simulink model "malt_pos_hold"  (R2023a)
settings: Solver=FixedStepAuto  StartTime=0.0  StopTime=50  FixedStep=framePeriod_s  RelTol=1e-3
undefined symbols (not defined in the file or in its folder): Aircraft, DiscIntNeverNeededParam, framePeriod_s, frameRate_hz
libraries: simulink x33, slpidlib x12
(part 2 of 3)

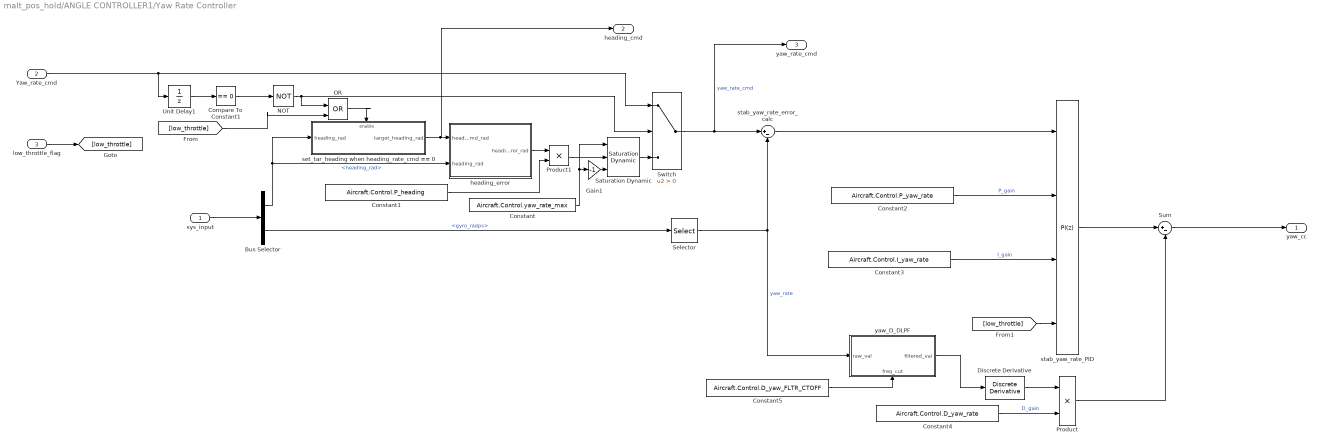
== system malt_pos_hold/ANGLE CONTROLLER1/Yaw Rate Controller ==
  sys_input : Inport
  Yaw_rate_cmd : Inport  Port=2
  low_throttle_flag : Inport  Port=3
  Bus Selector : BusSelector  OutputSignals=StateEstData.bfs_ins.heading_rad,StateEstData.bfs_ins.gyro_radps
  Compare To Constant1 : simulink/Logic and Bit Operations/Compare To Constant  relop===  const=0  OutDataTypeStr=boolean
  Constant : Constant  Value=Aircraft.Control.yaw_rate_max
  Constant1 : Constant  Value=Aircraft.Control.P_heading  OutDataTypeStr=single
  Constant2 : Constant  Value=Aircraft.Control.P_yaw_rate  OutDataTypeStr=single
  Constant3 : Constant  Value=Aircraft.Control.I_yaw_rate  OutDataTypeStr=single
  Constant4 : Constant  Value=Aircraft.Control.D_yaw_rate  OutDataTypeStr=single
  Constant5 : Constant  Value=Aircraft.Control.D_yaw_FLTR_CTOFF  OutDataTypeStr=single
  Discrete Derivative : simulink/Quick Insert/Discrete/Discrete Derivative  gainval=1.0  ICPrevScaledInput=0.0  OutMin=[]  OutMax=[]  OutDataType=fixdt(1, 16)  OutScaling=2^-10  DoSatur=off
  Gain1 : Gain  Gain=-1
  NOT : Logic  Operator=NOT  IconShape=distinctive  AllPortsSameDT=off  OutDataTypeStr=boolean
  OR : Logic  Operator=OR  IconShape=distinctive  AllPortsSameDT=off  OutDataTypeStr=boolean
  Product : Product
  Product1 : Product
  Saturation Dynamic : simulink/Discontinuities/Saturation Dynamic  OutMin=[]  OutMax=[]  OutDataTypeStr=Inherit: Same as second input  OutDataType=fixdt(1, 16)  OutScaling=2^-10  DoSatur=off
  Selector : Selector  InputPortWidth=3  IndexOptions=Index vector (dialog)  Indices=3  OutputSizes=1
  Sum : Sum  Inputs=|+-
  Switch : Switch  Criteria=u2 > Threshold  SaturateOnIntegerOverflow=off  InputSameDT=off
  Unit Delay1 : UnitDelay  InitialCondition=0.5  SampleTime=-1  HasFrameUpgradeWarning=on
  heading_error : Subsystem
  set_tar_heading when heading_rate_cmd == 0 : Subsystem  TreatAsAtomicUnit=on
  stab_yaw_rate_PID : slpidlib/PID Controller  Controller=PI  Form=Parallel  TimeDomain=Discrete-time  UseExternalTs=off  SampleTime=framePeriod_s  IntegratorMethod=Forward Euler  FilterMethod=Forward Euler  ControllerParametersSource=external  P=1.85  I=0.01  UseKiTs=off  D=0  N=100  UseFilter=off  TunerSelectOption=Transfer Function Based (PID Tuner App)  InitialConditionSource=internal  InitialConditionForIntegrator=0  InitialConditionForFilter=0  DifferentiatorICPrevScaledInput=0  ExternalReset=either  TrackingMode=off  Kt=1  LimitOutput=on  SatLimitsSource=internal  UpperSaturationLimit=1  LowerSaturationLimit=-1  LinearizeAsGain=off  AntiWindupMode=clamping  Kb=1  LimitIntegrator=off  UpperIntegratorSaturationLimit=inf  LowerIntegratorSaturationLimit=-inf  POutMin=[]  POutMax=[]  IOutMin=[]  IOutMax=[]  DOutMin=[]  DOutMax=[]  NOutMin=[]  NOutMax=[]  SumOutMin=[]  SumOutMax=[]  SaturationOutMin=[]  SaturationOutMax=[]  PParamMin=[]  PParamMax=[]  IParamMin=[]  IParamMax=[]  DParamMin=[]  DParamMax=[]  NParamMin=[]  NParamMax=[]  KbParamMin=[]  KbParamMax=[]  KtParamMin=[]  KtParamMax=[]  KbOutMin=[]  KbOutMax=[]  KtOutMin=[]  KtOutMax=[]  IntegratorOutMin=[]  IntegratorOutMax=[]  FilterOutMin=[]  FilterOutMax=[]  SumI1OutMin=[]  SumI1OutMax=[]  SumI2OutMin=[]  SumI2OutMax=[]  SumI3OutMin=[]  SumI3OutMax=[]  SumI4OutMin=[]  SumI4OutMax=[]  SumDOutMin=[]  SumDOutMax=[]  DifferentiatorOutMin=[]  DifferentiatorOutMax=[]  FilterDiffOutCoefMin=[]  FilterDiffOutCoefMax=[]  ReciprocalOutMin=[]  ReciprocalOutMax=[]  SumDenOutMin=[]  SumDenOutMax=[]  SumNumOutMin=[]  SumNumOutMax=[]  DivideOutMin=[]  DivideOutMax=[]  UdiffTsProdOutMin=[]  UdiffTsProdOutMax=[]  NTsProdOutMin=[]  NTsProdOutMax=[]  UintegralTsProdOutMin=[]  UintegralTsProdOutMax=[]  UngainTsProdOutMin=[]  UngainTsProdOutMax=[]  ClampingZeroOutDataTypeStr=Inherit: Inherit via back propagation  ClampingZeroOutMin=[]  ClampingZeroOutMax=[]  FilterDenConstantOutDataTypeStr=Inherit: Inherit via back propagation  FilterDenConstantOutMin=[]  FilterDenConstantOutMax=[]  PCopyOutDataTypeStr=Inherit: Inherit via back propagation  PCopyOutMin=[]  PCopyOutMax=[]  NCopyOutDataTypeStr=Inherit: Inherit via back propagation  NCopyOutMin=[]  NCopyOutMax=[]  IntegratorContinuousStateAttributes=''  IntegratorStateMustResolveToSignalObject=off  IntegratorRTWStateStorageClass=Auto  FilterContinuousStateAttributes=''  FilterStateMustResolveToSignalObject=off  FilterRTWStateStorageClass=Auto  ParallelPVariant=ExternalParameters  IdealPVariant=Disabled  IVariant=ExternalParameters  DVariant=Disabled  IntegratorVariant=Discrete  SatVariant=Enabled  AWVariant=DiscClampingParallel  PCopyVariant=Disabled  TRVariant=Disabled  FdbkBlocksVariant=Forward  IdealPFdbkVariant=Disabled  SatFdbkVariant=Disabled  DerivativeFilterVariant=Disabled  NVariant=Disabled  NCopyVariant=Disabled_SignalSpec  FilterICVariant=Disabled  IntegratorICVariant=InternalICs  ExternalResetVariant=ExternalReset  TRSumVariant=Passthrough  SumFdbkVariant=Disabled  SumVariant=Sum_PI  TsampFilterVariant=InternalTs  TsampNgainVariant=Passthrough  TsampIntegralVariant=Disabled_SignalSpec  ExternalSaturationOutDataTypeStr=Inherit: Same as second input
  stab_yaw_rate_error_calc : Sum  Inputs=|+-
  yaw_D_DLPF : Subsystem
      settings: PortSchema="{\"entries\":[{\"content\":{\"sides\":[{\"content\":{\"connectorIds\":[\"In1\"]},\"type\":\"ConnectorPlacement.EquallySpacedRectSide\",\"uuid\":\"20236834-aeb3-4c5b-bb2e-f84447e752b5\"},{\"content\":{\"connectorIds\":[\"Out1\"],\"side\":\"RIGHT\"},\"type\":\"ConnectorPlacement.EquallySpacedRectSide\",\"uuid\":\"d668f9a1-a3df-4207-8bf1-99fb838e59b2\"},{\"content\":{\"connectorIds\":[],\"side\":\"TOP\"},\"type\":\"ConnectorPlacement.EquallySpacedRectSide\",\"uuid\":\"66cceb06-f4bc-4278-b965-2427292e46df\"},{\"content\":{\"connectorIds\":[\"In2\"],\"side\":\"BOTTOM\"},\"type\":\"ConnectorPlacement.EquallySpacedRectSide\",\"uuid\":\"8fdaac6a-cb03-4bd4-87bb-7bafd10bc297\"}]},\"type\":\"ConnectorPlacement.EquallySpacedConnector\",\"uuid\":\"3dc29a9a-e794-478d-b7df-452e6c2d3f66\"}],\"packageUris\":[\"http://schema.mathworks.com/mf0/Connector/R2020b\"],\"version\":\"1.0\"}"
  yaw_cc : Outport
  heading_cmd : Outport  Port=2
  yaw_rate_cmd : Outport  Port=3
  wires:
  sys_input/1 -> Bus Selector/1
  Bus Selector/2 -> Selector/1  "<gyro_radps>"
  stab_yaw_rate_PID/1 -> Sum/1
  Sum/1 -> yaw_cc/1
  Product/1 -> Sum/2
  Discrete Derivative/1 -> Product/1
  Constant2/1 -> stab_yaw_rate_PID/2  "P_gain"
  Constant3/1 -> stab_yaw_rate_PID/3  "I_gain"
  Constant4/1 -> Product/2  "D_gain"
  Selector/1 -> stab_yaw_rate_error_calc/2, yaw_D_DLPF/1(raw_val)  "yaw_rate"
  Bus Selector/1 -> set_tar_heading when heading_rate_cmd == 0/1(heading_rad), heading_error/2(heading_rad)  "<heading_rad>"
  Switch/1 -> yaw_rate_cmd/1, stab_yaw_rate_error_calc/1  "yaw_rate_cmd"
  Yaw_rate_cmd/1 -> Unit Delay1/1, Switch/1
  heading_error/1(heading_error_rad) -> Product1/1
  Constant1/1 -> Product1/2
  set_tar_heading when heading_rate_cmd == 0/1(target_heading_rad) -> heading_cmd/1, heading_error/1(heading_cmd_rad)
  Product1/1 -> Saturation Dynamic/2
  Saturation Dynamic/1 -> Switch/3
  Gain1/1 -> Saturation Dynamic/3
  Constant/1 -> Saturation Dynamic/1, Gain1/1
  Constant5/1 -> yaw_D_DLPF/2(freq_cut)
  yaw_D_DLPF/1(filtered_val) -> Discrete Derivative/1
  stab_yaw_rate_error_calc/1 -> stab_yaw_rate_PID/1
  Unit Delay1/1 -> Compare To Constant1/1
  low_throttle_flag/1 -> [low_throttle]
  [low_throttle] -> OR/2
  NOT/1 -> Switch/2, OR/1
  Compare To Constant1/1 -> NOT/1
  [low_throttle] -> stab_yaw_rate_PID/4
  OR/1 -> set_tar_heading when heading_rate_cmd == 0/Enable

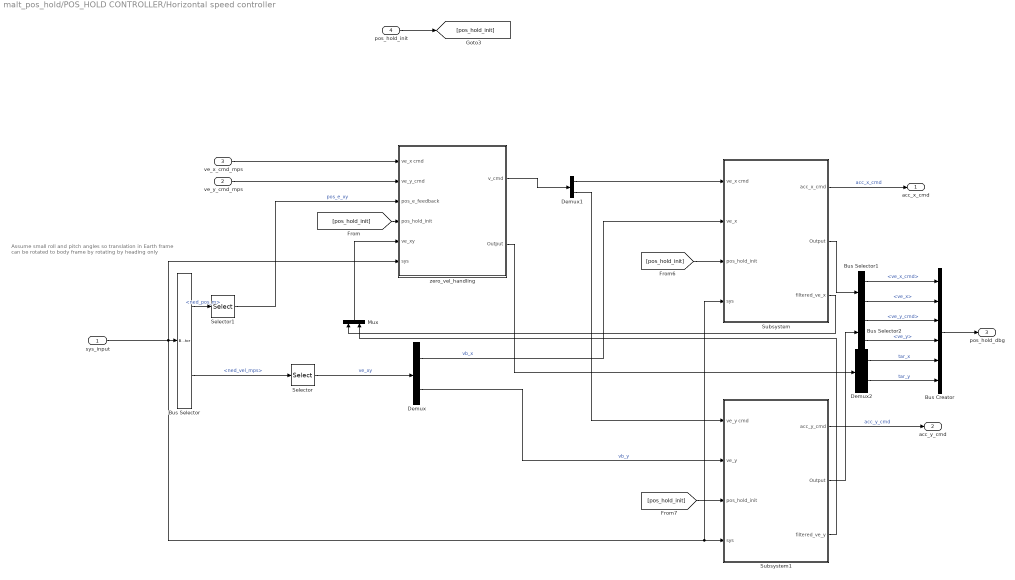
== system malt_pos_hold/POS_HOLD CONTROLLER/Horizontal speed controller ==
  note: Assume small roll and pitch angles so translation in Earth frame can be rotated to body frame by rotating by heading only
  sys_input : Inport
  ve_y_cmd_mps : Inport  Port=2
  ve_x_cmd_mps : Inport  Port=3
  pos_hold_init : Inport  Port=4
  Bus Creator : BusCreator  Inputs=6
  Bus Selector : BusSelector  OutputSignals=StateEstData.aux_ins.ned_pos_m,StateEstData.bfs_ins.ned_vel_mps
  Bus Selector1 : BusSelector  OutputSignals=ve_x_cmd,ve_x
  Bus Selector2 : BusSelector  OutputSignals=ve_y_cmd,ve_y
  Demux : Demux  Outputs=2
  Demux1 : Demux  Outputs=2
  Demux2 : Demux  Outputs=2
  Mux : Mux  Inputs=2
  Selector : Selector  InputPortWidth=3  IndexOptions=Index vector (dialog)  Indices=[1 2]  OutputSizes=1
  Selector1 : Selector  InputPortWidth=3  IndexOptions=Index vector (dialog)  Indices=[1 2]  OutputSizes=1
  Subsystem : Subsystem
  Subsystem1 : Subsystem
  zero_vel_handling : Subsystem
  acc_x_cmd : Outport
  acc_y_cmd : Outport  Port=2
  pos_hold_dbg : Outport  Port=3
  wires:
  Subsystem1/1(acc_y_cmd) -> acc_y_cmd/1  "acc_y_cmd"
  Subsystem/1(acc_x_cmd) -> acc_x_cmd/1  "acc_x_cmd"
  sys_input/1 -> Bus Selector/1, Subsystem/4(sys), Subsystem1/4(sys), zero_vel_handling/6(sys)
  Bus Selector/2 -> Selector/1  "<ned_vel_mps>"
  Demux/1 -> Subsystem/2(ve_x)  "vb_x"
  pos_hold_init/1 -> [pos_hold_init]
  [pos_hold_init] -> Subsystem/3(pos_hold_init)
  [pos_hold_init] -> Subsystem1/3(pos_hold_init)
  Subsystem/2(Output) -> Bus Selector1/1
  Subsystem1/2(Output) -> Bus Selector2/1
  Bus Selector1/1 -> Bus Creator/1  "<ve_x_cmd>"
  Bus Selector1/2 -> Bus Creator/2  "<ve_x>"
  Bus Selector2/1 -> Bus Creator/3  "<ve_y_cmd>"
  Bus Selector2/2 -> Bus Creator/4  "<ve_y>"
  Bus Creator/1 -> pos_hold_dbg/1
  Bus Selector/1 -> Selector1/1  "<ned_pos_m>"
  Demux/2 -> Subsystem1/2(ve_y)  "vb_y"
  ve_x_cmd_mps/1 -> zero_vel_handling/1(ve_x cmd)
  ve_y_cmd_mps/1 -> zero_vel_handling/2(ve_y_cmd)
  Selector1/1 -> zero_vel_handling/3(pos_e_feedback)  "pos_e_xy"
  [pos_hold_init] -> zero_vel_handling/4(pos_hold_init)
  zero_vel_handling/1(v_cmd) -> Demux1/1
  Demux1/1 -> Subsystem/1(ve_x cmd)
  Demux1/2 -> Subsystem1/1(ve_y cmd)
  zero_vel_handling/2(Output) -> Demux2/1
  Demux2/1 -> Bus Creator/5  "tar_x"
  Demux2/2 -> Bus Creator/6  "tar_y"
  Selector/1 -> Demux/1  "ve_xy"
  Subsystem/3(filtered_ve_x) -> Mux/1
  Subsystem1/3(filtered_ve_y) -> Mux/2
  Mux/1 -> zero_vel_handling/5(ve_xy)

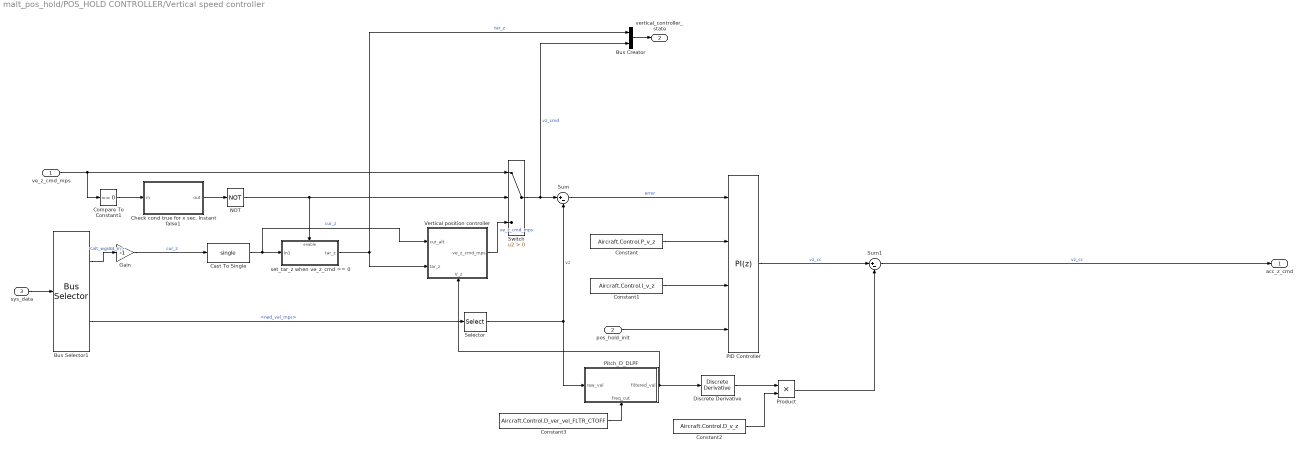
== system malt_pos_hold/POS_HOLD CONTROLLER/Vertical speed controller ==
  ve_z_cmd_mps : Inport
  pos_hold_init : Inport  Port=2
  sys_data : Inport  Port=3
  Bus Creator : BusCreator  Inputs=2
  Bus Selector1 : BusSelector  OutputSignals=StateEstData.bfs_ins.alt_wgs84_m,StateEstData.bfs_ins.ned_vel_mps
  Cast To Single : DataTypeConversion  OutDataTypeStr=single  SaturateOnIntegerOverflow=off  RndMeth=Floor
  Check cond true for x sec. Instant false1 : Subsystem
  Compare To Constant1 : simulink/Logic and Bit Operations/Compare To Constant  relop===  const=0  OutDataTypeStr=boolean
  Constant : Constant  Value=Aircraft.Control.P_v_z  OutDataTypeStr=single  SampleTime=framePeriod_s
  Constant1 : Constant  Value=Aircraft.Control.I_v_z  OutDataTypeStr=single  SampleTime=framePeriod_s
  Constant2 : Constant  Value=Aircraft.Control.D_v_z  OutDataTypeStr=single  SampleTime=framePeriod_s
  Constant3 : Constant  Value=Aircraft.Control.D_ver_vel_FLTR_CTOFF  OutDataTypeStr=single  SampleTime=framePeriod_s
  Discrete Derivative : simulink/Discrete/Discrete Derivative  gainval=1.0  ICPrevScaledInput=0.0  OutMin=[]  OutMax=[]  OutDataType=fixdt(1, 16)  OutScaling=2^-10  DoSatur=off
  Gain : Gain  Gain=-1
  NOT : Logic  Operator=NOT  IconShape=distinctive  AllPortsSameDT=off  OutDataTypeStr=boolean
  PID Controller : slpidlib/PID Controller  Controller=PI  Form=Parallel  TimeDomain=Discrete-time  UseExternalTs=off  SampleTime=framePeriod_s  IntegratorMethod=Forward Euler  FilterMethod=Forward Euler  ControllerParametersSource=external  P=0  I=0  UseKiTs=off  D=0  N=100  UseFilter=off  TunerSelectOption=Frequency Response Based  InitialConditionSource=internal  InitialConditionForIntegrator=0  InitialConditionForFilter=0  DifferentiatorICPrevScaledInput=0  ExternalReset=either  TrackingMode=off  Kt=1  LimitOutput=on  SatLimitsSource=internal  UpperSaturationLimit=1  LowerSaturationLimit=-1  LinearizeAsGain=on  AntiWindupMode=clamping  Kb=1  LimitIntegrator=off  UpperIntegratorSaturationLimit=inf  LowerIntegratorSaturationLimit=-inf  POutMin=[]  POutMax=[]  IOutMin=[]  IOutMax=[]  DOutMin=[]  DOutMax=[]  NOutMin=[]  NOutMax=[]  SumOutMin=[]  SumOutMax=[]  SaturationOutMin=[]  SaturationOutMax=[]  PParamMin=[]  PParamMax=[]  IParamMin=[]  IParamMax=[]  DParamMin=[]  DParamMax=[]  NParamMin=[]  NParamMax=[]  KbParamMin=[]  KbParamMax=[]  KtParamMin=[]  KtParamMax=[]  KbOutMin=[]  KbOutMax=[]  KtOutMin=[]  KtOutMax=[]  IntegratorOutMin=[]  IntegratorOutMax=[]  FilterOutMin=[]  FilterOutMax=[]  SumI1OutMin=[]  SumI1OutMax=[]  SumI2OutMin=[]  SumI2OutMax=[]  SumI3OutMin=[]  SumI3OutMax=[]  SumI4OutMin=[]  SumI4OutMax=[]  SumDOutMin=[]  SumDOutMax=[]  DifferentiatorOutMin=[]  DifferentiatorOutMax=[]  FilterDiffOutCoefMin=[]  FilterDiffOutCoefMax=[]  ReciprocalOutMin=[]  ReciprocalOutMax=[]  SumDenOutMin=[]  SumDenOutMax=[]  SumNumOutMin=[]  SumNumOutMax=[]  DivideOutMin=[]  DivideOutMax=[]  UdiffTsProdOutMin=[]  UdiffTsProdOutMax=[]  NTsProdOutMin=[]  NTsProdOutMax=[]  UintegralTsProdOutMin=[]  UintegralTsProdOutMax=[]  UngainTsProdOutMin=[]  UngainTsProdOutMax=[]  ClampingZeroOutDataTypeStr=Inherit: Inherit via back propagation  ClampingZeroOutMin=[]  ClampingZeroOutMax=[]  FilterDenConstantOutDataTypeStr=Inherit: Inherit via back propagation  FilterDenConstantOutMin=[]  FilterDenConstantOutMax=[]  PCopyOutDataTypeStr=Inherit: Inherit via back propagation  PCopyOutMin=[]  PCopyOutMax=[]  NCopyOutDataTypeStr=Inherit: Inherit via back propagation  NCopyOutMin=[]  NCopyOutMax=[]  IntegratorContinuousStateAttributes=''  IntegratorStateMustResolveToSignalObject=off  IntegratorRTWStateStorageClass=Auto  FilterContinuousStateAttributes=''  FilterStateMustResolveToSignalObject=off  FilterRTWStateStorageClass=Auto  ParallelPVariant=ExternalParameters  IdealPVariant=Disabled  IVariant=ExternalParameters  DVariant=Disabled  IntegratorVariant=Discrete  SatVariant=Enabled  AWVariant=DiscClampingParallel  PCopyVariant=Disabled  TRVariant=Disabled  FdbkBlocksVariant=Forward  IdealPFdbkVariant=Disabled  SatFdbkVariant=Disabled  DerivativeFilterVariant=Disabled  NVariant=Disabled  NCopyVariant=Disabled_SignalSpec  FilterICVariant=Disabled  IntegratorICVariant=InternalICs  ExternalResetVariant=ExternalReset  TRSumVariant=Passthrough  SumFdbkVariant=Disabled  SumVariant=Sum_PI  TsampFilterVariant=InternalTs  TsampNgainVariant=Passthrough  TsampIntegralVariant=Disabled_SignalSpec  ExternalSaturationOutDataTypeStr=Inherit: Same as second input
  Pitch_D_DLPF : Subsystem
      settings: PortSchema="{\"entries\":[{\"content\":{\"sides\":[{\"content\":{\"connectorIds\":[\"In1\"]},\"type\":\"ConnectorPlacement.EquallySpacedRectSide\",\"uuid\":\"20236834-aeb3-4c5b-bb2e-f84447e752b5\"},{\"content\":{\"connectorIds\":[\"Out1\"],\"side\":\"RIGHT\"},\"type\":\"ConnectorPlacement.EquallySpacedRectSide\",\"uuid\":\"d668f9a1-a3df-4207-8bf1-99fb838e59b2\"},{\"content\":{\"connectorIds\":[],\"side\":\"TOP\"},\"type\":\"ConnectorPlacement.EquallySpacedRectSide\",\"uuid\":\"66cceb06-f4bc-4278-b965-2427292e46df\"},{\"content\":{\"connectorIds\":[\"In2\"],\"side\":\"BOTTOM\"},\"type\":\"ConnectorPlacement.EquallySpacedRectSide\",\"uuid\":\"7d08bc25-8e2d-44c6-8f94-b04e75c70268\"}]},\"type\":\"ConnectorPlacement.EquallySpacedConnector\",\"uuid\":\"3dc29a9a-e794-478d-b7df-452e6c2d3f66\"}],\"packageUris\":[\"http://schema.mathworks.com/mf0/Connector/R2020b\"],\"version\":\"1.0\"}"
  Product : Product
  Selector : Selector  InputPortWidth=3  IndexOptions=Index vector (dialog)  Indices=[3]  OutputSizes=1
  Sum : Sum  Inputs=|+-
  Sum1 : Sum  Inputs=|+-
  Switch : Switch  Criteria=u2 > Threshold  SaturateOnIntegerOverflow=off  InputSameDT=off
  Vertical position controller : Subsystem
      settings: PortSchema="{\"entries\":[{\"content\":{\"sides\":[{\"content\":{\"connectorIds\":[\"In1\",\"In2\"]},\"type\":\"ConnectorPlacement.EquallySpacedRectSide\",\"uuid\":\"79520bb7-3b73-4b0a-afa5-00212f0d5535\"},{\"content\":{\"connectorIds\":[\"Out1\"],\"side\":\"RIGHT\"},\"type\":\"ConnectorPlacement.EquallySpacedRectSide\",\"uuid\":\"7af35bc0-787d-4ae6-9de8-6e73ac6b2f05\"},{\"content\":{\"side\":\"TOP\"},\"type\":\"ConnectorPlacement.EquallySpacedRectSide\",\"uuid\":\"9c439c94-e639-4f06-896e-953805e3ca95\"},{\"content\":{\"connectorIds\":[\"In3\"],\"side\":\"BOTTOM\"},\"type\":\"ConnectorPlacement.EquallySpacedRectSide\",\"uuid\":\"1da903b3-cd2c-46f1-9f19-ae5eef6857d5\"}]},\"type\":\"ConnectorPlacement.EquallySpacedConnector\",\"uuid\":\"f3f40da9-9611-4a13-b171-f91ff073ebb5\"}],\"packageUris\":[\"http://schema.mathworks.com/mf0/Connector/R2020b\"],\"version\":\"1.0\"}"
  set_tar_z when ve_z_cmd == 0 : Subsystem  TreatAsAtomicUnit=on
  acc_z_cmd : Outport
  vertical_controller_state : Outport  Port=2
  wires:
  Constant/1 -> PID Controller/2
  Bus Selector1/2 -> Selector/1  "<ned_vel_mps>"
  sys_data/1 -> Bus Selector1/1
  Pitch_D_DLPF/1(filtered_val) -> Vertical position controller/3(V_z), Discrete Derivative/1
  Selector/1 -> Sum/2, Pitch_D_DLPF/1(raw_val)  "vz"
  Constant2/1 -> Product/2
  Product/1 -> Sum1/2
  ve_z_cmd_mps/1 -> Switch/1, Compare To Constant1/1
  Compare To Constant1/1 -> Check cond true for x sec. Instant false1/1(in)
  Switch/1 -> Bus Creator/2, Sum/1  "vz_cmd"
  set_tar_z when ve_z_cmd == 0/1(tar_z) -> Bus Creator/1, Vertical position controller/2(tar_z)  "tar_z"
  pos_hold_init/1 -> PID Controller/4
  Constant3/1 -> Pitch_D_DLPF/2(freq_cut)
  Cast To Single/1 -> Vertical position controller/1(cur_alt), set_tar_z when ve_z_cmd == 0/1(In1)  "cur_z"
  Sum/1 -> PID Controller/1  "error"
  Sum1/1 -> acc_z_cmd/1  "vz_cc"
  PID Controller/1 -> Sum1/1  "vz_cc"
  Constant1/1 -> PID Controller/3
  Vertical position controller/1(ve_z_cmd_mps) -> Switch/3  "ve_z_cmd_mps"
  NOT/1 -> Switch/2, set_tar_z when ve_z_cmd == 0/Enable
  Bus Selector1/1 -> Gain/1  "<alt_wgs84_m>"
  Check cond true for x sec. Instant false1/1(out) -> NOT/1
  Gain/1 -> Cast To Single/1  "cur_z"
  Bus Creator/1 -> vertical_controller_state/1
  Discrete Derivative/1 -> Product/1

== system malt_pos_hold/POS_HOLD_input_conversion/body_to_inertial conversion ==
  vb_xy : Inport
  heading_rad : Inport  Port=2
  2D rotation from NED_xy to body_xy : Subsystem
  Demux : Demux  Outputs=2
  Product : Product  Multiplication=Matrix(*)
  Transpose : Math  Operator=transpose
  ve_x : Outport
  ve_y : Outport  Port=2
  wires:
  Demux/1 -> ve_x/1  "ve_x"
  Product/1 -> Demux/1  "ve_xy"
  heading_rad/1 -> 2D rotation from NED_xy to body_xy/1(<heading_rad>)
  vb_xy/1 -> Product/2
  2D rotation from NED_xy to body_xy/1(2D_rot) -> Transpose/1
  Demux/2 -> ve_y/1  "ve_y"
  Transpose/1 -> Product/1

== system malt_pos_hold/POS_HOLD_input_conversion/pitch_norm_deadband ==
  raw_sbus_in : Inport
  deadband : Inport  Port=2
  Constant : Constant  Value=0  OutDataTypeStr=single
  Constant1 : Constant  Value=Aircraft.Control.v_z_max  OutDataTypeStr=single
  Constant2 : Constant  Value=-Aircraft.Control.v_z_max  OutDataTypeStr=single
  Constant3 : Constant  OutDataTypeStr=single
  remap_with_deadband : MATLAB Function  TreatAsAtomicUnit=on
  normalized_out : Outport
  wires:
  deadband/1 -> remap_with_deadband/6(deadband)
  Constant2/1 -> remap_with_deadband/5(out_max)
  Constant1/1 -> remap_with_deadband/4(out_min)
  Constant3/1 -> remap_with_deadband/3(in_max)
  Constant/1 -> remap_with_deadband/2(in_min)
  remap_with_deadband/1(norm_out) -> normalized_out/1
  raw_sbus_in/1 -> remap_with_deadband/1(raw_in)

== system malt_pos_hold/Stab_input_conversion/remap from min_spin to max ==
  raw_in : Inport
  Constant4 : Constant  Value=0  OutDataTypeStr=single
  Constant5 : Constant  Value=Aircraft.Control.motor_spin_min  OutDataTypeStr=single
  Constant6 : Constant  OutDataTypeStr=single
  Constant7 : Constant  OutDataTypeStr=single
  remap1 : MATLAB Function  TreatAsAtomicUnit=on
  norm_out : Outport
  wires:
  Constant6/1 -> remap1/5(out_max)
  Constant5/1 -> remap1/4(out_min)
  remap1/1(norm_out) -> norm_out/1
  Constant4/1 -> remap1/2(in_min)
  Constant7/1 -> remap1/3(in_max)
  raw_in/1 -> remap1/1(raw_in)

== system malt_pos_hold/cmd to raw pwm1/motor_PWM_denormalize ==
  normalized_input : Inport
  Constant : Constant  Value=0  OutDataTypeStr=single
  Constant1 : Constant  Value=1100  OutDataTypeStr=single
  Constant2 : Constant  Value=1950  OutDataTypeStr=single
  Constant3 : Constant  OutDataTypeStr=single
  remap : MATLAB Function  TreatAsAtomicUnit=on
  raw_output : Outport
  wires:
  Constant2/1 -> remap/5(out_max)
  Constant1/1 -> remap/4(out_min)
  Constant3/1 -> remap/3(in_max)
  Constant/1 -> remap/2(in_min)
  remap/1(raw_out) -> raw_output/1
  normalized_input/1 -> remap/1(norm_in)

== system malt_pos_hold/command selection/e_stop_norm ==
  raw_sbus_in : Inport
  Constant : Constant  Value=172  OutDataTypeStr=single
  Constant1 : Constant  Value=-1  OutDataTypeStr=single
  Constant2 : Constant  OutDataTypeStr=single
  Constant3 : Constant  Value=1811  OutDataTypeStr=single
  remap : MATLAB Function  TreatAsAtomicUnit=on
  normalized_out : Outport
  wires:
  Constant2/1 -> remap/5(out_max)
  Constant1/1 -> remap/4(out_min)
  Constant3/1 -> remap/3(in_max)
  Constant/1 -> remap/2(in_min)
  remap/1(norm_out) -> normalized_out/1
  raw_sbus_in/1 -> remap/1(raw_in)

== system malt_pos_hold/command selection/mode_norm ==
  raw_sbus_in : Inport
  Constant : Constant  Value=172  OutDataTypeStr=single
  Constant1 : Constant  Value=0  OutDataTypeStr=single
  Constant2 : Constant  Value=2  OutDataTypeStr=single
  Constant3 : Constant  Value=1811  OutDataTypeStr=single
  remap : MATLAB Function  TreatAsAtomicUnit=on
  normalized_out : Outport
  wires:
  raw_sbus_in/1 -> remap/1(raw_in)
  remap/1(norm_out) -> normalized_out/1
  Constant/1 -> remap/2(in_min)
  Constant3/1 -> remap/3(in_max)
  Constant1/1 -> remap/4(out_min)
  Constant2/1 -> remap/5(out_max)

== system malt_pos_hold/command selection/mode_norm1 ==
  raw_sbus_in : Inport
  Constant : Constant  Value=172  OutDataTypeStr=single
  Constant1 : Constant  Value=0  OutDataTypeStr=single
  Constant2 : Constant  OutDataTypeStr=single
  Constant3 : Constant  Value=1811  OutDataTypeStr=single
  remap : MATLAB Function  TreatAsAtomicUnit=on
  normalized_out : Outport
  wires:
  Constant2/1 -> remap/5(out_max)
  Constant1/1 -> remap/4(out_min)
  Constant3/1 -> remap/3(in_max)
  Constant/1 -> remap/2(in_min)
  remap/1(norm_out) -> normalized_out/1
  raw_sbus_in/1 -> remap/1(raw_in)

== system malt_pos_hold/command selection/pitch_norm_deadband ==
  raw_sbus_in : Inport
  deadband : Inport  Port=2
  Constant : Constant  Value=172  OutDataTypeStr=single
  Constant1 : Constant  Value=-1  OutDataTypeStr=single
  Constant2 : Constant  OutDataTypeStr=single
  Constant3 : Constant  Value=1811  OutDataTypeStr=single
  remap_with_deadband : MATLAB Function  TreatAsAtomicUnit=on
  normalized_out : Outport
  wires:
  deadband/1 -> remap_with_deadband/6(deadband)
  Constant2/1 -> remap_with_deadband/5(out_max)
  Constant1/1 -> remap_with_deadband/4(out_min)
  Constant3/1 -> remap_with_deadband/3(in_max)
  Constant/1 -> remap_with_deadband/2(in_min)
  remap_with_deadband/1(norm_out) -> normalized_out/1
  raw_sbus_in/1 -> remap_with_deadband/1(raw_in)

== system malt_pos_hold/command selection/roll_norm_deadband ==
  raw_sbus_in : Inport
  deadband : Inport  Port=2
  Constant : Constant  Value=172  OutDataTypeStr=single
  Constant1 : Constant  Value=-1  OutDataTypeStr=single
  Constant2 : Constant  OutDataTypeStr=single
  Constant3 : Constant  Value=1811  OutDataTypeStr=single
  remap_with_deadband : MATLAB Function  TreatAsAtomicUnit=on
  normalized_out : Outport
  wires:
  deadband/1 -> remap_with_deadband/6(deadband)
  Constant2/1 -> remap_with_deadband/5(out_max)
  Constant1/1 -> remap_with_deadband/4(out_min)
  Constant3/1 -> remap_with_deadband/3(in_max)
  Constant/1 -> remap_with_deadband/2(in_min)
  remap_with_deadband/1(norm_out) -> normalized_out/1
  raw_sbus_in/1 -> remap_with_deadband/1(raw_in)

== system malt_pos_hold/command selection/throttle_norm ==
  raw_sbus_in : Inport
  Constant : Constant  Value=172  OutDataTypeStr=single
  Constant1 : Constant  Value=0  OutDataTypeStr=single
  Constant2 : Constant  OutDataTypeStr=single
  Constant3 : Constant  Value=1811  OutDataTypeStr=single
  remap : MATLAB Function  TreatAsAtomicUnit=on
  normalized_out : Outport
  wires:
  raw_sbus_in/1 -> remap/1(raw_in)
  remap/1(norm_out) -> normalized_out/1
  Constant/1 -> remap/2(in_min)
  Constant3/1 -> remap/3(in_max)
  Constant1/1 -> remap/4(out_min)
  Constant2/1 -> remap/5(out_max)

== system malt_pos_hold/command selection/yaw_norm_deadband ==
  raw_sbus_in : Inport
  deadband : Inport  Port=2
  Constant : Constant  Value=172  OutDataTypeStr=single
  Constant1 : Constant  Value=-1  OutDataTypeStr=single
  Constant2 : Constant  OutDataTypeStr=single
  Constant3 : Constant  Value=1811  OutDataTypeStr=single
  remap_with_deadband : MATLAB Function  TreatAsAtomicUnit=on
  normalized_out : Outport
  wires:
  raw_sbus_in/1 -> remap_with_deadband/1(raw_in)
  remap_with_deadband/1(norm_out) -> normalized_out/1
  Constant/1 -> remap_with_deadband/2(in_min)
  Constant3/1 -> remap_with_deadband/3(in_max)
  Constant1/1 -> remap_with_deadband/4(out_min)
  Constant2/1 -> remap_with_deadband/5(out_max)
  deadband/1 -> remap_with_deadband/6(deadband)

== system malt_pos_hold/determine arm and mode selection/Failsafe_management ==
  note: - radio failsafe
  In Bus Element1 : Inport  PortName=inceptor  Element=failsafe
  manual_mode : Inport  Port=2
  motor_state : Inport  Port=3
  NOT : Logic  Operator=NOT  IconShape=distinctive  AllPortsSameDT=off  OutDataTypeStr=boolean
  Radio failsafe : Subsystem
  radio_failsafe_enabled : Outport
  wires:
  Radio failsafe/1(radio_failsafe_enabled) -> radio_failsafe_enabled/1
  manual_mode/1 -> Radio failsafe/2(manual_mode)
  motor_state/1 -> Radio failsafe/3(motor_state)
  In Bus Element1/1 -> NOT/1
  NOT/1 -> Radio failsafe/1(failsafe)

== system malt_pos_hold/determine arm and mode selection/Subsystem ==
  <e_stop> : Inport
  Abs1 : Abs  SaturateOnIntegerOverflow=off
  Compare To Constant : simulink/Logic and Bit Operations/Compare To Constant  relop=>=  const=0.98  OutDataTypeStr=boolean
  e_stop counter : Subsystem
  e_stop_filtered : Outport
  wires:
  Compare To Constant/1 -> e_stop counter/Enable
  Abs1/1 -> Compare To Constant/1
  <e_stop>/1 -> e_stop counter/1(motor_e_stop_raw), Abs1/1
  e_stop counter/1(e_stop_filtered) -> e_stop_filtered/1

== system malt_pos_hold/determine arm and mode selection/yaw_stick_arming ==
  note: yaw_stick arming
  <yaw> : Inport
  <throttle> : Inport  Port=2
  e_stop : Inport  Port=3
  AND : Logic  IconShape=distinctive  AllPortsSameDT=off  OutDataTypeStr=boolean
  Abs : Abs  SaturateOnIntegerOverflow=off
  Cast To Single : DataTypeConversion  OutDataTypeStr=single  SaturateOnIntegerOverflow=off  RndMeth=Floor
  Compare To Constant : simulink/Logic and Bit Operations/Compare To Constant  relop=>  const=0  OutDataTypeStr=boolean
  Compare To Constant1 : simulink/Logic and Bit Operations/Compare To Constant  relop=>=  const=0.95  OutDataTypeStr=boolean
  Compare To Constant2 : simulink/Logic and Bit Operations/Compare To Constant  relop=>=  const=3  OutDataTypeStr=boolean
  Compare To Constant3 : simulink/Logic and Bit Operations/Compare To Constant  relop=<=  const=0.03  OutDataTypeStr=boolean
  Compare To Constant4 : simulink/Logic and Bit Operations/Compare To Constant  relop=>=  const=0.5  OutDataTypeStr=boolean
  Constant : Constant  Value=0  OutDataTypeStr=boolean  LockScale=on
  Enabled Subsystem : Subsystem  TreatAsAtomicUnit=on
  OR : Logic  Operator=OR  IconShape=distinctive  AllPortsSameDT=off  OutDataTypeStr=boolean
  Sum : Sum  Inputs=-+|
  Switch : Switch  Criteria=u2 > Threshold  SaturateOnIntegerOverflow=off  InputSameDT=off
  Unit Delay : UnitDelay  SampleTime=-1  HasFrameUpgradeWarning=on
  manual_arming : Subsystem
  arm_state : Outport
  wires:
  Enabled Subsystem/1(time_arm_valid_s) -> Compare To Constant2/1
  Abs/1 -> Compare To Constant1/1
  Compare To Constant1/1 -> AND/2, Enabled Subsystem/1(yaw_input)
  Compare To Constant4/1 -> manual_arming/1(yaw_arm)
  AND/1 -> Enabled Subsystem/Enable
  <yaw>/1 -> Compare To Constant4/1, Abs/1
  <throttle>/1 -> Compare To Constant3/1
  Compare To Constant3/1 -> AND/1
  Constant/1 -> Switch/1
  manual_arming/1(arm_state) -> Switch/3
  Switch/1 -> arm_state/1
  e_stop/1 -> OR/1, Switch/2
  OR/1 -> manual_arming/Trigger
  Compare To Constant2/1 -> Cast To Single/1
  Sum/1 -> Compare To Constant/1
  Unit Delay/1 -> Sum/1
  Cast To Single/1 -> Unit Delay/1, Sum/2
  Compare To Constant/1 -> OR/2

== system malt_pos_hold/ANGLE CONTROLLER1/Pitch Controller/pitch_D_DLPF ==
  raw_val : Inport
  freq_cut : Inport  Port=2
  Constant : Constant  Value=frameRate_hz  OutDataTypeStr=single
  MATLAB Function : MATLAB Function  TreatAsAtomicUnit=on
  Unit Delay : UnitDelay  SampleTime=-1  HasFrameUpgradeWarning=on
  filtered_val : Outport
  wires:
  freq_cut/1 -> MATLAB Function/3(freq_cut)
  MATLAB Function/1(filtered_val) -> Unit Delay/1, filtered_val/1
  Unit Delay/1 -> MATLAB Function/1(prev_val)
  raw_val/1 -> MATLAB Function/2(raw_val)
  Constant/1 -> MATLAB Function/4(samp_freq)

== system malt_pos_hold/ANGLE CONTROLLER1/Roll Controller/roll_D_DLPF ==
  raw_val : Inport
  freq_cut : Inport  Port=2
  Constant : Constant  Value=frameRate_hz  OutDataTypeStr=single
  MATLAB Function : MATLAB Function  TreatAsAtomicUnit=on
  Unit Delay : UnitDelay  SampleTime=-1  HasFrameUpgradeWarning=on
  filtered_val : Outport
  wires:
  freq_cut/1 -> MATLAB Function/3(freq_cut)
  MATLAB Function/1(filtered_val) -> Unit Delay/1, filtered_val/1
  Unit Delay/1 -> MATLAB Function/1(prev_val)
  raw_val/1 -> MATLAB Function/2(raw_val)
  Constant/1 -> MATLAB Function/4(samp_freq)

== system malt_pos_hold/ANGLE CONTROLLER1/Yaw Rate Controller/heading_error ==
  heading_cmd_rad : Inport
  heading_rad : Inport  Port=2
  Abs : Abs  SaturateOnIntegerOverflow=off
  Compare To Constant : simulink/Logic and Bit Operations/Compare To Constant  relop=>  const=pi  OutDataTypeStr=boolean
  Constant : Constant  Value=2*pi  OutDataTypeStr=single
  Constant1 : Constant  Value=4.712391  OutDataTypeStr=single
  Product : Product
  Sign : Signum
  Subtract : Sum  Inputs=+-
  Subtract1 : Sum  Inputs=+-
  Switch : Switch  Criteria=u2 > Threshold  SaturateOnIntegerOverflow=off  InputSameDT=off
  heading_error_rad : Outport
  wires:
  heading_rad/1 -> Subtract/2
  Subtract/1 -> Abs/1, Switch/3, Subtract1/1, Sign/1
  Compare To Constant/1 -> Switch/2
  Subtract1/1 -> Switch/1
  Switch/1 -> heading_error_rad/1
  Abs/1 -> Compare To Constant/1
  Sign/1 -> Product/1
  Product/1 -> Subtract1/2
  Constant/1 -> Product/2
  Constant1/1 -> Subtract/1

== system malt_pos_hold/ANGLE CONTROLLER1/Yaw Rate Controller/set_tar_heading when heading_rate_cmd == 0 ==
  heading_rad : Inport
  Enable : EnablePort
  target_heading_rad : Outport
  wires:
  heading_rad/1 -> target_heading_rad/1

== system malt_pos_hold/ANGLE CONTROLLER1/Yaw Rate Controller/yaw_D_DLPF ==
  raw_val : Inport
  freq_cut : Inport  Port=2
  Constant : Constant  Value=frameRate_hz  OutDataTypeStr=single
  MATLAB Function : MATLAB Function  TreatAsAtomicUnit=on
  Unit Delay : UnitDelay  SampleTime=-1  HasFrameUpgradeWarning=on
  filtered_val : Outport
  wires:
  freq_cut/1 -> MATLAB Function/3(freq_cut)
  MATLAB Function/1(filtered_val) -> Unit Delay/1, filtered_val/1
  Unit Delay/1 -> MATLAB Function/1(prev_val)
  raw_val/1 -> MATLAB Function/2(raw_val)
  Constant/1 -> MATLAB Function/4(samp_freq)

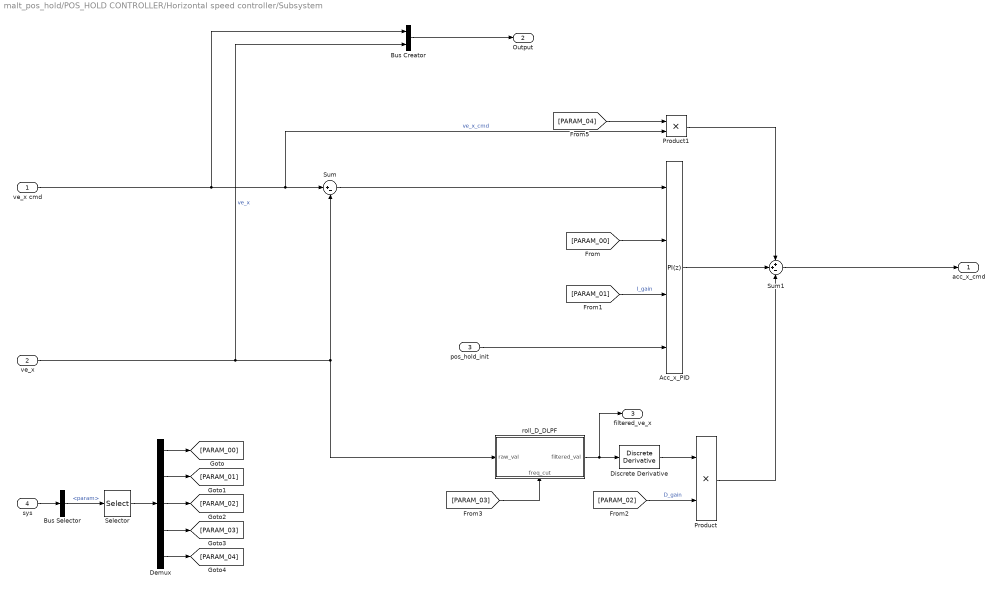
== system malt_pos_hold/POS_HOLD CONTROLLER/Horizontal speed controller/Subsystem ==
  ve_x cmd : Inport
  ve_x : Inport  Port=2
  pos_hold_init : Inport  Port=3
  sys : Inport  Port=4
  Acc_x_PID : slpidlib/PID Controller  Controller=PI  Form=Parallel  TimeDomain=Discrete-time  UseExternalTs=off  SampleTime=framePeriod_s  IntegratorMethod=Forward Euler  FilterMethod=Forward Euler  ControllerParametersSource=external  P=0.335  I=0.005  UseKiTs=off  D=0  N=100  UseFilter=off  TunerSelectOption=Transfer Function Based (PID Tuner App)  InitialConditionSource=internal  InitialConditionForIntegrator=0  InitialConditionForFilter=0  DifferentiatorICPrevScaledInput=0  ExternalReset=either  TrackingMode=off  Kt=1  LimitOutput=off  SatLimitsSource=internal  UpperSaturationLimit=Aircraft.Control.pitch_angle_lim  LowerSaturationLimit=-Aircraft.Control.pitch_angle_lim  LinearizeAsGain=off  AntiWindupMode=clamping  Kb=1  LimitIntegrator=off  UpperIntegratorSaturationLimit=inf  LowerIntegratorSaturationLimit=-inf  POutMin=[]  POutMax=[]  IOutMin=[]  IOutMax=[]  DOutMin=[]  DOutMax=[]  NOutMin=[]  NOutMax=[]  SumOutMin=[]  SumOutMax=[]  SaturationOutMin=[]  SaturationOutMax=[]  PParamMin=[]  PParamMax=[]  IParamMin=[]  IParamMax=[]  DParamMin=[]  DParamMax=[]  NParamMin=[]  NParamMax=[]  KbParamMin=[]  KbParamMax=[]  KtParamMin=[]  KtParamMax=[]  KbOutMin=[]  KbOutMax=[]  KtOutMin=[]  KtOutMax=[]  IntegratorOutMin=[]  IntegratorOutMax=[]  FilterOutMin=[]  FilterOutMax=[]  SumI1OutMin=[]  SumI1OutMax=[]  SumI2OutMin=[]  SumI2OutMax=[]  SumI3OutMin=[]  SumI3OutMax=[]  SumI4OutMin=[]  SumI4OutMax=[]  SumDOutMin=[]  SumDOutMax=[]  DifferentiatorOutMin=[]  DifferentiatorOutMax=[]  FilterDiffOutCoefMin=[]  FilterDiffOutCoefMax=[]  ReciprocalOutMin=[]  ReciprocalOutMax=[]  SumDenOutMin=[]  SumDenOutMax=[]  SumNumOutMin=[]  SumNumOutMax=[]  DivideOutMin=[]  DivideOutMax=[]  UdiffTsProdOutMin=[]  UdiffTsProdOutMax=[]  NTsProdOutMin=[]  NTsProdOutMax=[]  UintegralTsProdOutMin=[]  UintegralTsProdOutMax=[]  UngainTsProdOutMin=[]  UngainTsProdOutMax=[]  ClampingZeroOutDataTypeStr=Inherit: Inherit via back propagation  ClampingZeroOutMin=[]  ClampingZeroOutMax=[]  FilterDenConstantOutDataTypeStr=Inherit: Inherit via back propagation  FilterDenConstantOutMin=[]  FilterDenConstantOutMax=[]  PCopyOutDataTypeStr=Inherit: Inherit via back propagation  PCopyOutMin=[]  PCopyOutMax=[]  NCopyOutDataTypeStr=Inherit: Inherit via back propagation  NCopyOutMin=[]  NCopyOutMax=[]  IntegratorContinuousStateAttributes=''  IntegratorStateMustResolveToSignalObject=off  IntegratorRTWStateStorageClass=Auto  FilterContinuousStateAttributes=''  FilterStateMustResolveToSignalObject=off  FilterRTWStateStorageClass=Auto  ParallelPVariant=ExternalParameters  IdealPVariant=Disabled  IVariant=ExternalParameters  DVariant=Disabled  IntegratorVariant=Discrete  SatVariant=Disabled  AWVariant=Passthrough  PCopyVariant=Disabled  TRVariant=Disabled  FdbkBlocksVariant=Forward  IdealPFdbkVariant=Disabled  SatFdbkVariant=Disabled  DerivativeFilterVariant=Disabled  NVariant=Disabled  NCopyVariant=Disabled_SignalSpec  FilterICVariant=Disabled  IntegratorICVariant=InternalICs  ExternalResetVariant=ExternalReset  TRSumVariant=Passthrough  SumFdbkVariant=Disabled  SumVariant=Sum_PI  TsampFilterVariant=InternalTs  TsampNgainVariant=Passthrough  TsampIntegralVariant=Disabled_SignalSpec  ExternalSaturationOutDataTypeStr=Inherit: Same as second input
  Bus Creator : BusCreator  Inputs=2
  Bus Selector : BusSelector  OutputSignals=Telemetry Data.param
  Demux : Demux  Outputs=5
  Discrete Derivative : simulink/Discrete/Discrete Derivative  gainval=1.0  ICPrevScaledInput=0.0  OutMin=[]  OutMax=[]  OutDataType=fixdt(1, 16)  OutScaling=2^-10  DoSatur=off
  Product : Product
  Product1 : Product
  Selector : Selector  IndexMode=Zero-based  InputPortWidth=24  IndexOptions=Index vector (dialog)  Indices=[0 1 2 3 4]  OutputSizes=1
  Sum : Sum  Inputs=|+-
  Sum1 : Sum  Inputs=++-
  roll_D_DLPF : Subsystem
      settings: PortSchema="{\"entries\":[{\"content\":{\"sides\":[{\"content\":{\"connectorIds\":[\"In1\"]},\"type\":\"ConnectorPlacement.EquallySpacedRectSide\",\"uuid\":\"20236834-aeb3-4c5b-bb2e-f84447e752b5\"},{\"content\":{\"connectorIds\":[\"Out1\"],\"side\":\"RIGHT\"},\"type\":\"ConnectorPlacement.EquallySpacedRectSide\",\"uuid\":\"d668f9a1-a3df-4207-8bf1-99fb838e59b2\"},{\"content\":{\"connectorIds\":[],\"side\":\"TOP\"},\"type\":\"ConnectorPlacement.EquallySpacedRectSide\",\"uuid\":\"66cceb06-f4bc-4278-b965-2427292e46df\"},{\"content\":{\"connectorIds\":[\"In2\"],\"side\":\"BOTTOM\"},\"type\":\"ConnectorPlacement.EquallySpacedRectSide\",\"uuid\":\"8fdaac6a-cb03-4bd4-87bb-7bafd10bc297\"}]},\"type\":\"ConnectorPlacement.EquallySpacedConnector\",\"uuid\":\"3dc29a9a-e794-478d-b7df-452e6c2d3f66\"}],\"packageUris\":[\"http://schema.mathworks.com/mf0/Connector/R2020b\"],\"version\":\"1.0\"}"
  acc_x_cmd : Outport
  Output : Outport  Port=2
  filtered_ve_x : Outport  Port=3
  wires:
  ve_x/1 -> Bus Creator/2, roll_D_DLPF/1(raw_val), Sum/2  "ve_x"
  Sum/1 -> Acc_x_PID/1
  [PARAM_00] -> Acc_x_PID/2
  [PARAM_01] -> Acc_x_PID/3  "I_gain"
  pos_hold_init/1 -> Acc_x_PID/4
  [PARAM_02] -> Product/2  "D_gain"
  Discrete Derivative/1 -> Product/1
  [PARAM_03] -> roll_D_DLPF/2(freq_cut)
  roll_D_DLPF/1(filtered_val) -> filtered_ve_x/1, Discrete Derivative/1
  Bus Creator/1 -> Output/1
  ve_x cmd/1 -> Product1/2, Sum/1, Bus Creator/1  "ve_x_cmd"
  Sum1/1 -> acc_x_cmd/1
  sys/1 -> Bus Selector/1
  Bus Selector/1 -> Selector/1  "<param>"
  Selector/1 -> Demux/1
  Demux/1 -> [PARAM_00]
  Demux/3 -> [PARAM_02]
  Demux/2 -> [PARAM_01]
  Demux/4 -> [PARAM_03]
  Demux/5 -> [PARAM_04]
  [PARAM_04] -> Product1/1
  Product1/1 -> Sum1/1
  Acc_x_PID/1 -> Sum1/2
  Product/1 -> Sum1/3

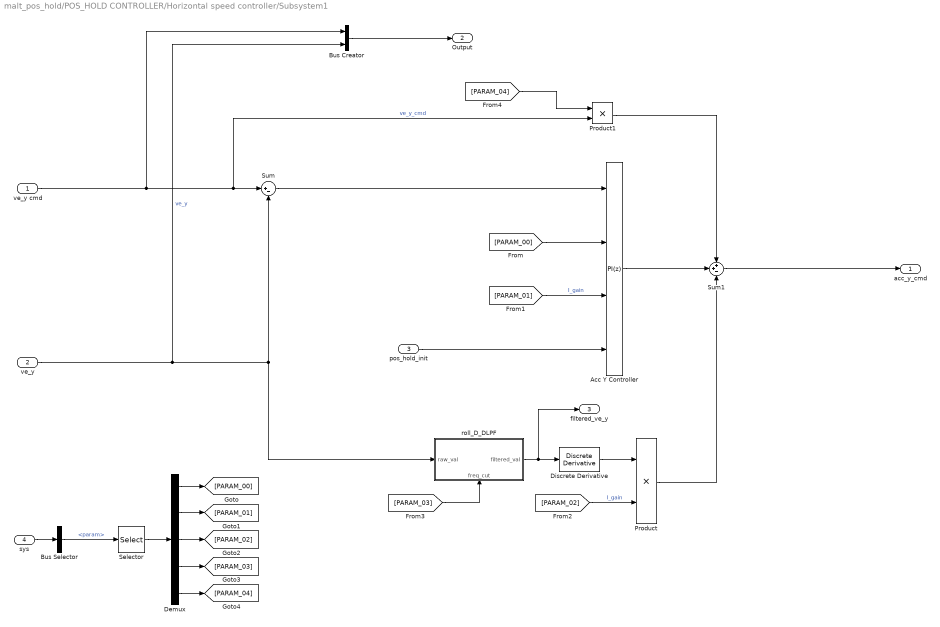
== system malt_pos_hold/POS_HOLD CONTROLLER/Horizontal speed controller/Subsystem1 ==
  ve_y cmd : Inport
  ve_y : Inport  Port=2
  pos_hold_init : Inport  Port=3
  sys : Inport  Port=4
  Acc Y Controller : slpidlib/PID Controller  Controller=PI  Form=Parallel  TimeDomain=Discrete-time  UseExternalTs=off  SampleTime=framePeriod_s  IntegratorMethod=Forward Euler  FilterMethod=Forward Euler  ControllerParametersSource=external  P=0.335  I=0.005  UseKiTs=off  D=0  N=100  UseFilter=off  TunerSelectOption=Transfer Function Based (PID Tuner App)  InitialConditionSource=internal  InitialConditionForIntegrator=0  InitialConditionForFilter=0  DifferentiatorICPrevScaledInput=0  ExternalReset=either  TrackingMode=off  Kt=1  LimitOutput=off  SatLimitsSource=internal  UpperSaturationLimit=Aircraft.Control.roll_angle_lim  LowerSaturationLimit=-Aircraft.Control.roll_angle_lim  LinearizeAsGain=off  AntiWindupMode=clamping  Kb=1  LimitIntegrator=on  UpperIntegratorSaturationLimit=4  LowerIntegratorSaturationLimit=-4  POutMin=[]  POutMax=[]  IOutMin=[]  IOutMax=[]  DOutMin=[]  DOutMax=[]  NOutMin=[]  NOutMax=[]  SumOutMin=[]  SumOutMax=[]  SaturationOutMin=[]  SaturationOutMax=[]  PParamMin=[]  PParamMax=[]  IParamMin=[]  IParamMax=[]  DParamMin=[]  DParamMax=[]  NParamMin=[]  NParamMax=[]  KbParamMin=[]  KbParamMax=[]  KtParamMin=[]  KtParamMax=[]  KbOutMin=[]  KbOutMax=[]  KtOutMin=[]  KtOutMax=[]  IntegratorOutMin=[]  IntegratorOutMax=[]  FilterOutMin=[]  FilterOutMax=[]  SumI1OutMin=[]  SumI1OutMax=[]  SumI2OutMin=[]  SumI2OutMax=[]  SumI3OutMin=[]  SumI3OutMax=[]  SumI4OutMin=[]  SumI4OutMax=[]  SumDOutMin=[]  SumDOutMax=[]  DifferentiatorOutMin=[]  DifferentiatorOutMax=[]  FilterDiffOutCoefMin=[]  FilterDiffOutCoefMax=[]  ReciprocalOutMin=[]  ReciprocalOutMax=[]  SumDenOutMin=[]  SumDenOutMax=[]  SumNumOutMin=[]  SumNumOutMax=[]  DivideOutMin=[]  DivideOutMax=[]  UdiffTsProdOutMin=[]  UdiffTsProdOutMax=[]  NTsProdOutMin=[]  NTsProdOutMax=[]  UintegralTsProdOutMin=[]  UintegralTsProdOutMax=[]  UngainTsProdOutMin=[]  UngainTsProdOutMax=[]  ClampingZeroOutDataTypeStr=Inherit: Inherit via back propagation  ClampingZeroOutMin=[]  ClampingZeroOutMax=[]  FilterDenConstantOutDataTypeStr=Inherit: Inherit via back propagation  FilterDenConstantOutMin=[]  FilterDenConstantOutMax=[]  PCopyOutDataTypeStr=Inherit: Inherit via back propagation  PCopyOutMin=[]  PCopyOutMax=[]  NCopyOutDataTypeStr=Inherit: Inherit via back propagation  NCopyOutMin=[]  NCopyOutMax=[]  IntegratorContinuousStateAttributes=''  IntegratorStateMustResolveToSignalObject=off  IntegratorRTWStateStorageClass=Auto  FilterContinuousStateAttributes=''  FilterStateMustResolveToSignalObject=off  FilterRTWStateStorageClass=Auto  ParallelPVariant=ExternalParameters  IdealPVariant=Disabled  IVariant=ExternalParameters  DVariant=Disabled  IntegratorVariant=Discrete  SatVariant=Disabled  AWVariant=Passthrough  PCopyVariant=Disabled  TRVariant=Disabled  FdbkBlocksVariant=Forward  IdealPFdbkVariant=Disabled  SatFdbkVariant=Disabled  DerivativeFilterVariant=Disabled  NVariant=Disabled  NCopyVariant=Disabled_SignalSpec  FilterICVariant=Disabled  IntegratorICVariant=InternalICs  ExternalResetVariant=ExternalReset  TRSumVariant=Passthrough  SumFdbkVariant=Disabled  SumVariant=Sum_PI  TsampFilterVariant=InternalTs  TsampNgainVariant=Passthrough  TsampIntegralVariant=Disabled_SignalSpec  ExternalSaturationOutDataTypeStr=Inherit: Same as second input
  Bus Creator : BusCreator  Inputs=2
  Bus Selector : BusSelector  OutputSignals=Telemetry Data.param
  Demux : Demux  Outputs=5
  Discrete Derivative : simulink/Discrete/Discrete Derivative  gainval=1.0  ICPrevScaledInput=0.0  OutMin=[]  OutMax=[]  OutDataType=fixdt(1, 16)  OutScaling=2^-10  DoSatur=off
  Product : Product
  Product1 : Product
  Selector : Selector  IndexMode=Zero-based  InputPortWidth=24  IndexOptions=Index vector (dialog)  Indices=[0 1 2 3 4]  OutputSizes=1
  Sum : Sum  Inputs=|+-
  Sum1 : Sum  Inputs=++-
  roll_D_DLPF : Subsystem
      settings: PortSchema="{\"entries\":[{\"content\":{\"sides\":[{\"content\":{\"connectorIds\":[\"In1\"]},\"type\":\"ConnectorPlacement.EquallySpacedRectSide\",\"uuid\":\"20236834-aeb3-4c5b-bb2e-f84447e752b5\"},{\"content\":{\"connectorIds\":[\"Out1\"],\"side\":\"RIGHT\"},\"type\":\"ConnectorPlacement.EquallySpacedRectSide\",\"uuid\":\"d668f9a1-a3df-4207-8bf1-99fb838e59b2\"},{\"content\":{\"connectorIds\":[],\"side\":\"TOP\"},\"type\":\"ConnectorPlacement.EquallySpacedRectSide\",\"uuid\":\"66cceb06-f4bc-4278-b965-2427292e46df\"},{\"content\":{\"connectorIds\":[\"In2\"],\"side\":\"BOTTOM\"},\"type\":\"ConnectorPlacement.EquallySpacedRectSide\",\"uuid\":\"8fdaac6a-cb03-4bd4-87bb-7bafd10bc297\"}]},\"type\":\"ConnectorPlacement.EquallySpacedConnector\",\"uuid\":\"3dc29a9a-e794-478d-b7df-452e6c2d3f66\"}],\"packageUris\":[\"http://schema.mathworks.com/mf0/Connector/R2020b\"],\"version\":\"1.0\"}"
  acc_y_cmd : Outport
  Output : Outport  Port=2
  filtered_ve_y : Outport  Port=3
  wires:
  ve_y/1 -> Bus Creator/2, roll_D_DLPF/1(raw_val), Sum/2  "ve_y"
  Sum/1 -> Acc Y Controller/1
  Sum1/1 -> acc_y_cmd/1
  [PARAM_00] -> Acc Y Controller/2
  [PARAM_01] -> Acc Y Controller/3  "I_gain"
  pos_hold_init/1 -> Acc Y Controller/4
  Discrete Derivative/1 -> Product/1
  [PARAM_03] -> roll_D_DLPF/2(freq_cut)
  roll_D_DLPF/1(filtered_val) -> filtered_ve_y/1, Discrete Derivative/1
  Bus Creator/1 -> Output/1
  ve_y cmd/1 -> Product1/2, Sum/1, Bus Creator/1  "ve_y_cmd"
  [PARAM_02] -> Product/2  "I_gain"
  Bus Selector/1 -> Selector/1  "<param>"
  sys/1 -> Bus Selector/1
  [PARAM_04] -> Product1/1
  Acc Y Controller/1 -> Sum1/2
  Product/1 -> Sum1/3
  Product1/1 -> Sum1/1
  Demux/1 -> [PARAM_00]
  Demux/2 -> [PARAM_01]
  Demux/3 -> [PARAM_02]
  Demux/5 -> [PARAM_04]
  Selector/1 -> Demux/1
  Demux/4 -> [PARAM_03]

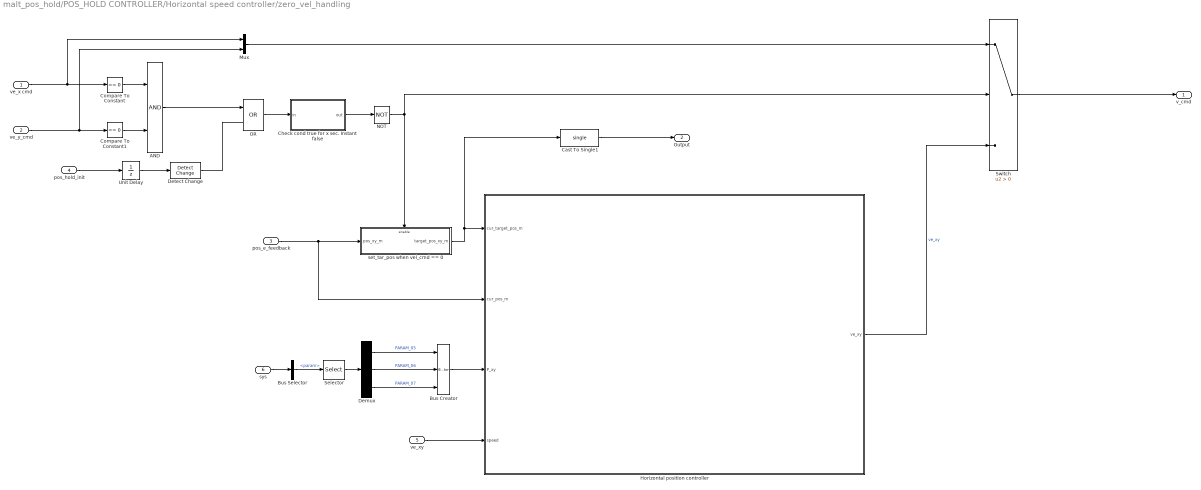
== system malt_pos_hold/POS_HOLD CONTROLLER/Horizontal speed controller/zero_vel_handling ==
  ve_x cmd : Inport
  ve_y_cmd : Inport  Port=2
  pos_e_feedback : Inport  Port=3
  pos_hold_init : Inport  Port=4
  ve_xy : Inport  Port=5
  sys : Inport  Port=6
  AND : Logic  IconShape=distinctive  AllPortsSameDT=off  OutDataTypeStr=boolean
  Bus Creator : BusCreator  Inputs=3
  Bus Selector : BusSelector  OutputSignals=Telemetry Data.param
  Cast To Single1 : DataTypeConversion  OutDataTypeStr=single  SaturateOnIntegerOverflow=off  RndMeth=Floor
  Check cond true for x sec. Instant false : Subsystem
  Compare To Constant : simulink/Logic and Bit Operations/Compare To Constant  relop===  const=0  OutDataTypeStr=boolean
  Compare To Constant1 : simulink/Logic and Bit Operations/Compare To Constant  relop===  const=0  OutDataTypeStr=boolean
  Demux : Demux  Outputs=3
  Detect Change : simulink/Logic and Bit Operations/Detect Change  vinit=0  OutDataTypeStr=boolean
  Horizontal position controller : Subsystem
  Mux : Mux  Inputs=2
  NOT : Logic  Operator=NOT  IconShape=distinctive  AllPortsSameDT=off  OutDataTypeStr=boolean
  OR : Logic  Operator=OR  IconShape=distinctive  AllPortsSameDT=off  OutDataTypeStr=boolean
  Selector : Selector  IndexMode=Zero-based  InputPortWidth=24  IndexOptions=Index vector (dialog)  Indices=[5 6 7]  OutputSizes=1
  Switch : Switch  Criteria=u2 > Threshold  SaturateOnIntegerOverflow=off  InputSameDT=off
  Unit Delay : UnitDelay  SampleTime=-1  HasFrameUpgradeWarning=on
  set_tar_pos when vel_cmd == 0 : Subsystem  TreatAsAtomicUnit=on
  v_cmd : Outport
  Output : Outport  Port=2
  wires:
  ve_y_cmd/1 -> Mux/2, Compare To Constant1/1
  Compare To Constant1/1 -> AND/2
  Switch/1 -> v_cmd/1
  ve_x cmd/1 -> Mux/1, Compare To Constant/1
  Compare To Constant/1 -> AND/1
  pos_e_feedback/1 -> set_tar_pos when vel_cmd == 0/1(pos_xy_m), Horizontal position controller/2(cur_pos_m)
  set_tar_pos when vel_cmd == 0/1(target_pos_xy_m) -> Cast To Single1/1, Horizontal position controller/1(cur_target_pos_m)
  OR/1 -> Check cond true for x sec. Instant false/1(in)
  AND/1 -> OR/1
  pos_hold_init/1 -> Unit Delay/1
  Detect Change/1 -> OR/2
  Unit Delay/1 -> Detect Change/1
  Cast To Single1/1 -> Output/1
  Bus Selector/1 -> Selector/1  "<param>"
  sys/1 -> Bus Selector/1
  Mux/1 -> Switch/1
  Horizontal position controller/1(ve_xy) -> Switch/3  "ve_xy"
  NOT/1 -> Switch/2, set_tar_pos when vel_cmd == 0/Enable
  Check cond true for x sec. Instant false/1(out) -> NOT/1
  Selector/1 -> Demux/1
  Demux/1 -> Bus Creator/1  "PARAM_05"
  Demux/2 -> Bus Creator/2  "PARAM_06"
  Demux/3 -> Bus Creator/3  "PARAM_07"
  Bus Creator/1 -> Horizontal position controller/3(P_xy)
  ve_xy/1 -> Horizontal position controller/4(speed)

== system malt_pos_hold/POS_HOLD CONTROLLER/Vertical speed controller/Check cond true for x sec. Instant false1 ==
  in : Inport
  Cast To Single : DataTypeConversion  OutDataTypeStr=single  SaturateOnIntegerOverflow=off  RndMeth=Floor
  Compare To time of signal true : simulink/Logic and Bit Operations/Compare To Constant  relop=>=  const=1  OutDataTypeStr=boolean
  Discrete-Time Integrator : DiscreteIntegrator  ExternalReset=falling  SampleTime=-1  ICPrevOutput=DiscIntNeverNeededParam  ICPrevScaledInput=DiscIntNeverNeededParam
  out : Outport
  wires:
  Compare To time of signal true/1 -> out/1
  in/1 -> Cast To Single/1, Discrete-Time Integrator/2
  Cast To Single/1 -> Discrete-Time Integrator/1
  Discrete-Time Integrator/1 -> Compare To time of signal true/1

== system malt_pos_hold/POS_HOLD CONTROLLER/Vertical speed controller/Pitch_D_DLPF ==
  raw_val : Inport
  freq_cut : Inport  Port=2
  MATLAB Function : MATLAB Function  TreatAsAtomicUnit=on
  Unit Delay : UnitDelay  SampleTime=-1  HasFrameUpgradeWarning=on
  filtered_val : Outport
  wires:
  MATLAB Function/1(filtered_val) -> filtered_val/1, Unit Delay/1
  raw_val/1 -> MATLAB Function/2(raw_val)
  Unit Delay/1 -> MATLAB Function/1(prev_val)
  freq_cut/1 -> MATLAB Function/3(freq_cut)
